simulink model "heli_model2"  (Simulink 10.3)
settings: Solver=ode1  StartTime=0.0  StopTime=100  FixedStep=0.001  RelTol=1e-3
values from neighbouring files (symbols this model uses):
  B_p = 0.0100000    (= 0.01)    [setup_heli_LQR_instructor.m]    (also in setup_heli_LQR_parameters.m)
  B_y = 0.0071428    [setup_heli_LQR_instructor.m]    (also in setup_heli_LQR_parameters.m)
  g = 9.81    [setup_heli_LQR_instructor.m]    (also in setup_heli_LQR_parameters.m)
  h = 0.0139    [setup_heli_LQR_instructor.m]    (also in setup_heli_LQR_parameters.m)
  J_eq_p = 0.0500    (= 0.05)    [setup_heli_LQR_instructor.m]    (also in setup_heli_LQR_parameters.m)
  J_eq_y = 0.0500+0.0039    (= 0.0539)    [setup_heli_LQR_instructor.m]    (also in setup_heli_LQR_parameters.m)
  K_pp = 0.185*0.20962    (= 0.0387797)    [setup_heli_LQR_instructor.m]    (also in setup_heli_LQR_parameters.m)
  K_py = 0.0041362    [setup_heli_LQR_instructor.m]    (also in setup_heli_LQR_parameters.m)
  K_yp = 0.0083316    [setup_heli_LQR_instructor.m]    (also in setup_heli_LQR_parameters.m)
  K_yy = 0.185*0.050271    (= 0.009300135)    [setup_heli_LQR_instructor.m]    (also in setup_heli_LQR_parameters.m)
  Ki = lqr(a,b,Qi,R)    [setup_heli_LQR_instructor.m]
  l_cm = 0.0168    [setup_heli_LQR_instructor.m]    (also in setup_heli_LQR_parameters.m)
  m_heli = 1.326    [setup_heli_LQR_instructor.m]    (also in setup_heli_LQR_parameters.m)
  Rc = 0.0094    [setup_heli_LQR_instructor.m]    (also in setup_heli_LQR_parameters.m)
  SAT_INT_ERR_PITCH = 20    [setup_heli_LQR_instructor.m]    (also in setup_heli_LQR_parameters.m)
  SAT_INT_ERR_YAW = 20    [setup_heli_LQR_instructor.m]    (also in setup_heli_LQR_parameters.m)
  theta_0 = -30*pi/180    (= -0.523598775598)    [setup_heli_LQR_instructor.m]    (also in setup_heli_LQR_parameters.m)
  Tr_p = 1    [setup_heli_LQR_instructor.m]    (also in setup_heli_LQR_parameters.m)
  Tr_y = 1    [setup_heli_LQR_instructor.m]    (also in setup_heli_LQR_parameters.m)
  VMAX_UPM_P = 24    [setup_heli_LQR_instructor.m]    (also in setup_heli_LQR_parameters.m)
  VMAX_UPM_Y = 15    [setup_heli_LQR_instructor.m]    (also in setup_heli_LQR_parameters.m)
undefined symbols (not defined in the file or in its folder): heli_2d_lib, Scopes
libraries: simulink_extras x4
settings Model: Creator=Joseph  LastModifiedBy=Joseph  ExtModeArmWhenConnect=off
settings DataIOCC: LimitDataPoints=on
settings OptimizationCC: BooleanDataType=off  OptimizeBlockIOStorage=off  BufferReuse=off  ExpressionFolding=off  ExpressionDepthLimit=128  LocalBlockOutputs=off  InitFltsAndDblsToZero=on
settings DebuggingCC: SaveWithParameterizedLinksMsg=none  SignalResolutionControl=TryResolveAllWithWarning  SolverPrmCheckMsg=warning  MultiTaskDSMMsg=warning  MultiTaskCondExecSysMsg=none  StateNameClashWarn=none
settings SFSimCC: SimUseLocalCustomCode=on  CustomCodeUndefinedFunction=FilterOut
settings RTWCC: Description=WinCon Target  SystemTargetFile=wincon.tlc  MakeCommand=make_wc  TemplateMakefile=wc_default_tmf  RTWUseLocalCustomCode=on
settings STFCustomTargetCC: TargetFcnLib=ansi_tfl_tmw.mat  ModelReferenceCompliant=off  CPPClassGenCompliant=on  SystemTargetFile=wincon.tlc
settings GRTTargetCC: TargetFcnLib=ansi_tfl_tmw.mat  ModelReferenceCompliant=off  ParMdlRefBuildCompliant=off  CompOptLevelCompliant=off  ConcurrentExecutionCompliant=off  MatFileLogging=off  UseToolchainInfoCompliant=off  ExtMode=on  ExtModeTransport=2  ExtModeMexFile=wc_comm
settings CustomProperty: Value=on
settings ConfigComp: CovExternalEMLEnable=on

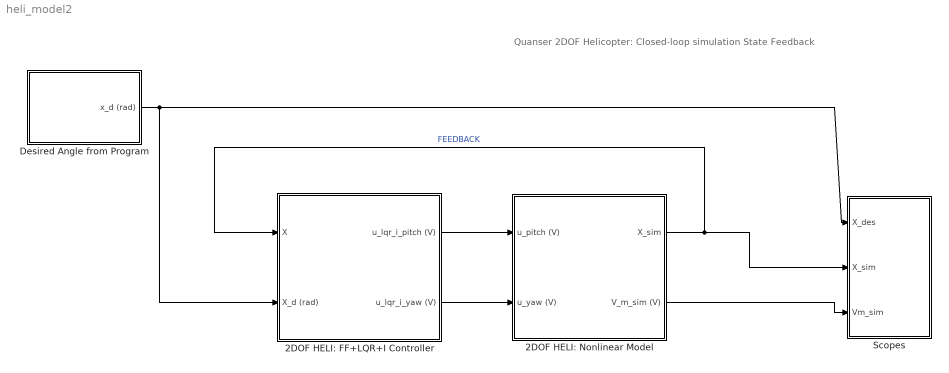
== system heli_model2 ==
  note: Quanser 2DOF Helicopter: Closed-loop simulation
      | State Feedback
  2DOF HELI: FF+LQR+I Controller : Subsystem  AncestorBlock=heli_2d_lib/2DOF HELI: FF+LQR+I Controller
  2DOF HELI: Nonlinear Model : Subsystem  AncestorBlock=heli_2d_lib/2DOF HELI: Nonlinear Model
  Desired Angle from Program : Subsystem
  Scopes : Subsystem  AncestorBlock=heli_2d_lib/Scopes
  wires:
  Desired Angle from Program/1(x_d (rad)) -> Scopes/1(X_des), 2DOF HELI: FF+LQR+I Controller/2(X_d (rad))
  2DOF HELI: FF+LQR+I Controller/1(u_lqr_i_pitch (V)) -> 2DOF HELI: Nonlinear Model/1(u_pitch (V))
  2DOF HELI: FF+LQR+I Controller/2(u_lqr_i_yaw (V)) -> 2DOF HELI: Nonlinear Model/2(u_yaw (V))
  2DOF HELI: Nonlinear Model/1(X_sim) -> Scopes/2(X_sim), 2DOF HELI: FF+LQR+I Controller/1(X)  "FEEDBACK"
  2DOF HELI: Nonlinear Model/2(V_m_sim (V)) -> Scopes/3(Vm_sim)

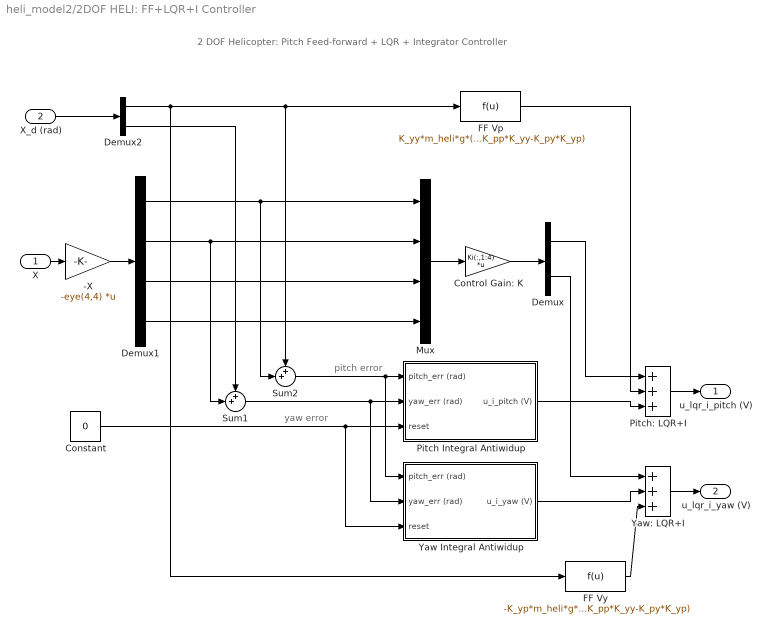
== system heli_model2/2DOF HELI: FF+LQR+I Controller ==
  note: yaw error
  note: pitch error
  note: 2 DOF Helicopter:
      | Pitch Feed-forward + LQR + Integrator Controller
  X : Inport
  X_d (rad) : Inport  Port=2
  -X : Gain  Gain=-eye(4,4)  Multiplication=Matrix(K*u)
  Constant : Constant  Value=0
  Control Gain: K : Gain  Gain=Ki(:,1:4)  Multiplication=Matrix(K*u)
  Demux : Demux  Outputs=2
  Demux1 : Demux
  Demux2 : Demux  Outputs=2
  FF Vp : Fcn  Expr="K_yy*m_heli*g*(h*sin(u[1]) + Rc*cos(u[1]))  /  (K_pp*K_yy-K_py*K_yp)"
  FF Vy : Fcn  Expr="-K_yp*m_heli*g*(h*sin(u[1]) + Rc*cos(u[1]))  /  (K_pp*K_yy-K_py*K_yp)"
  Mux : Mux
  Pitch Integral Antiwidup : Subsystem  AncestorBlock=heli_2d_lib/2DOF HELI: FF+LQR+I Controller/Yaw Integral Antiwidup
  Pitch: LQR+I : Sum  Inputs=+++
  Sum1 : Sum  Inputs=++|
  Sum2 : Sum  Inputs=++|
  Yaw Integral Antiwidup : Subsystem
  Yaw: LQR+I : Sum  Inputs=+++
  u_lqr_i_pitch (V) : Outport
  u_lqr_i_yaw (V) : Outport  Port=2
  wires:
  Constant/1 -> Pitch Integral Antiwidup/3(reset), Yaw Integral Antiwidup/3(reset)
  Demux1/2 -> Sum1/2, Mux/2
  Demux2/2 -> Sum1/1
  Demux2/1 -> Sum2/1, FF Vp/1, FF Vy/1
  X_d (rad)/1 -> Demux2/1
  Yaw Integral Antiwidup/1(u_i_yaw (V)) -> Yaw: LQR+I/2
  Demux/2 -> Yaw: LQR+I/1
  Yaw: LQR+I/1 -> u_lqr_i_yaw (V)/1
  Pitch: LQR+I/1 -> u_lqr_i_pitch (V)/1
  Demux/1 -> Pitch: LQR+I/2
  Pitch Integral Antiwidup/1(u_i_pitch (V)) -> Pitch: LQR+I/3
  FF Vp/1 -> Pitch: LQR+I/1
  Sum2/1 -> Pitch Integral Antiwidup/1(pitch_err (rad)), Yaw Integral Antiwidup/1(pitch_err (rad))
  Demux1/1 -> Sum2/2, Mux/1
  X/1 -> -X/1
  Sum1/1 -> Pitch Integral Antiwidup/2(yaw_err (rad)), Yaw Integral Antiwidup/2(yaw_err (rad))
  -X/1 -> Demux1/1
  Control Gain: K/1 -> Demux/1
  Mux/1 -> Control Gain: K/1
  Demux1/3 -> Mux/3
  Demux1/4 -> Mux/4
  FF Vy/1 -> Yaw: LQR+I/3

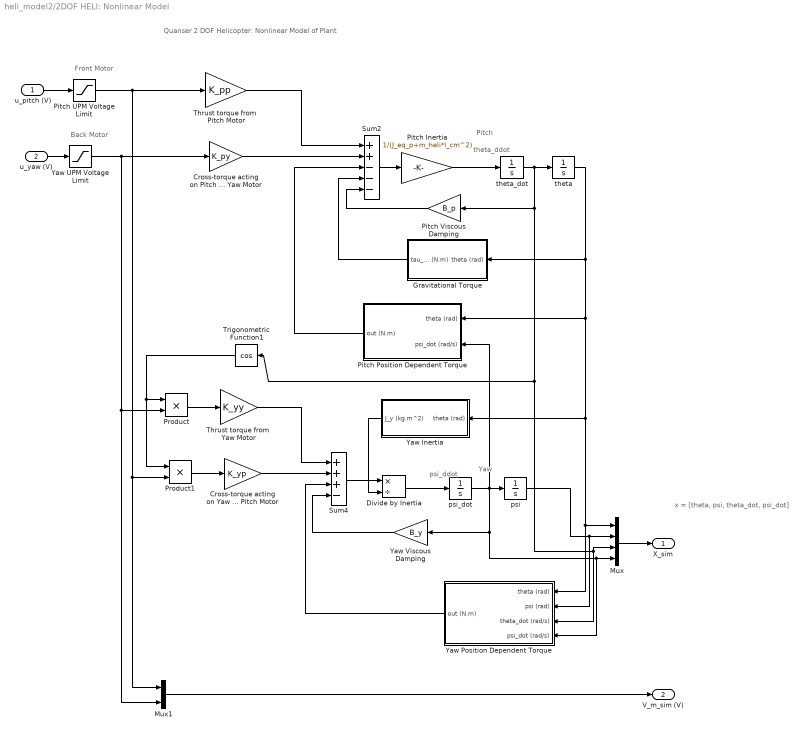
== system heli_model2/2DOF HELI: Nonlinear Model ==
  note: Back Motor
  note: Front Motor
  note: x = [theta, psi, theta_dot, psi_dot]
  note: Quanser 2 DOF Helicopter: Nonlinear Model of Plant
  note: theta_ddot
  note: psi_ddot
  note: Pitch
  note: Yaw
  u_pitch (V) : Inport
  u_yaw (V) : Inport  Port=2
  Cross-torque acting on Pitch  from Yaw Motor : Gain  Gain=K_py
  Cross-torque acting on Yaw  from Pitch Motor : Gain  Gain=K_yp
  Divide by Inertia : Product  Inputs=*/
  Gravitational Torque : Subsystem
  Mux : Mux
  Mux1 : Mux  Inputs=2
  Pitch Inertia : Gain  Gain=1/(J_eq_p+m_heli*l_cm^2)
  Pitch Position Dependent Torque : Subsystem  AncestorBlock=heli_2d_lib/2DOF Helicopter: Nonlinear Model/Yaw Nonlinear Element
  Pitch UPM Voltage Limit : Saturate  UpperLimit=VMAX_UPM_P  LowerLimit=- VMAX_UPM_P
  Pitch Viscous Damping : Gain  Gain=B_p
  Product : Product  RndMeth=Zero
  Product1 : Product  RndMeth=Zero
  Sum2 : Sum  Inputs=++---
  Sum4 : Sum  Inputs=+++-
  Thrust torque from  Pitch Motor : Gain  Gain=K_pp
  Thrust torque from  Yaw Motor : Gain  Gain=K_yy
  Trigonometric Function1 : Trigonometry  Operator=cos  OutputSignalType=real
  Yaw Inertia : Subsystem
  Yaw Position Dependent Torque : Subsystem
  Yaw UPM Voltage Limit : Saturate  UpperLimit=VMAX_UPM_Y  LowerLimit=- VMAX_UPM_Y
  Yaw Viscous Damping : Gain  Gain=B_y
  psi : Integrator
  psi_dot : Integrator
  theta : Integrator  InitialCondition=theta_0  LimitOutput=on  UpperSaturationLimit=40.5*pi/180  LowerSaturationLimit=-40.5*pi/180
  theta_dot : Integrator
  X_sim : Outport
  V_m_sim (V) : Outport  Port=2
  wires:
  Pitch Position Dependent Torque/1(out (N.m)) -> Sum2/3
  Gravitational Torque/1(tau_g (N.m)) -> Sum2/4
  Pitch Viscous Damping/1 -> Sum2/5
  Cross-torque acting on Pitch  from Yaw Motor/1 -> Sum2/2
  Thrust torque from  Pitch Motor/1 -> Sum2/1
  Yaw Inertia/1(J_y (kg.m^2)) -> Divide by Inertia/2
  Divide by Inertia/1 -> psi_dot/1
  Sum4/1 -> Divide by Inertia/1
  Yaw Position Dependent Torque/1(out (N.m)) -> Sum4/3
  Yaw Viscous Damping/1 -> Sum4/4
  psi/1 -> Yaw Position Dependent Torque/2(psi (rad)), Mux/2
  Mux1/1 -> V_m_sim (V)/1
  Yaw UPM Voltage Limit/1 -> Cross-torque acting on Pitch  from Yaw Motor/1, Mux1/2, Product/2
  Pitch UPM Voltage Limit/1 -> Thrust torque from  Pitch Motor/1, Mux1/1, Product1/2
  Mux/1 -> X_sim/1
  theta/1 -> Gravitational Torque/1(theta (rad)), Pitch Position Dependent Torque/1(theta (rad)), Yaw Position Dependent Torque/1(theta (rad)), Mux/1, Yaw Inertia/1(theta (rad))
  Sum2/1 -> Pitch Inertia/1
  Pitch Inertia/1 -> theta_dot/1
  theta_dot/1 -> Pitch Viscous Damping/1, Yaw Position Dependent Torque/3(theta_dot (rad/s)), Mux/3, Trigonometric Function1/1, theta/1
  Thrust torque from  Yaw Motor/1 -> Sum4/1
  Cross-torque acting on Yaw  from Pitch Motor/1 -> Sum4/2
  psi_dot/1 -> Yaw Viscous Damping/1, Yaw Position Dependent Torque/4(psi_dot (rad/s)), Mux/4, Pitch Position Dependent Torque/2(psi_dot (rad/s)), psi/1
  u_pitch (V)/1 -> Pitch UPM Voltage Limit/1
  u_yaw (V)/1 -> Yaw UPM Voltage Limit/1
  Product/1 -> Thrust torque from  Yaw Motor/1
  Trigonometric Function1/1 -> Product/1, Product1/1
  Product1/1 -> Cross-torque acting on Yaw  from Pitch Motor/1

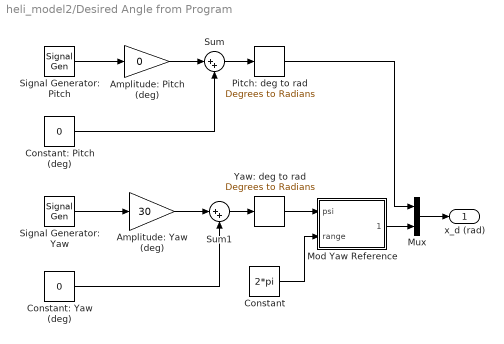
== system heli_model2/Desired Angle from Program ==
  Amplitude: Pitch (deg) : Gain  Gain=0
  Amplitude: Yaw (deg) : Gain  Gain=30
  Constant : Constant  Value=2*pi
  Constant: Pitch (deg) : Constant  Value=0
  Constant: Yaw (deg) : Constant  Value=0
  Mod Yaw Reference : Subsystem
  Mux : Mux  Inputs=2
  Pitch: deg to rad : simulink_extras/Transformations/Degrees to Radians
  Signal Generator: Pitch : SignalGenerator  WaveForm=square  Frequency=1/20
  Signal Generator: Yaw : SignalGenerator  WaveForm=square  Frequency=0.05
  Sum : Sum  Inputs=|++
  Sum1 : Sum  Inputs=|++
  Yaw: deg to rad : simulink_extras/Transformations/Degrees to Radians
  x_d (rad) : Outport
  wires:
  Mux/1 -> x_d (rad)/1
  Constant: Yaw (deg)/1 -> Sum1/2
  Amplitude: Yaw (deg)/1 -> Sum1/1
  Signal Generator: Yaw/1 -> Amplitude: Yaw (deg)/1
  Sum1/1 -> Yaw: deg to rad/1
  Constant: Pitch (deg)/1 -> Sum/2
  Amplitude: Pitch (deg)/1 -> Sum/1
  Signal Generator: Pitch/1 -> Amplitude: Pitch (deg)/1
  Sum/1 -> Pitch: deg to rad/1
  Pitch: deg to rad/1 -> Mux/1
  Mod Yaw Reference/1(mod psi) -> Mux/2
  Yaw: deg to rad/1 -> Mod Yaw Reference/1(psi)
  Constant/1 -> Mod Yaw Reference/2(range)

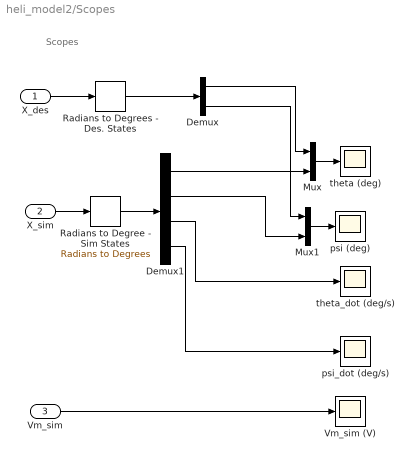
== system heli_model2/Scopes ==
  note: Scopes
  X_des : Inport
  X_sim : Inport  Port=2
  Vm_sim : Inport  Port=3
  Demux : Demux  Outputs=2
  Demux1 : Demux
  Mux : Mux  Inputs=2
  Mux1 : Mux  Inputs=2
  Radians to Degree - Sim States : simulink_extras/Transformations/Radians to Degrees
  Radians to Degrees - Des. States : simulink_extras/Transformations/Radians to Degrees
  Vm_sim (V) : Scope
  psi (deg) : Scope
  psi_dot (deg/s) : Scope
  theta (deg) : Scope
  theta_dot (deg/s) : Scope
  wires:
  Demux1/4 -> psi_dot (deg/s)/1
  Demux1/3 -> theta_dot (deg/s)/1
  Mux1/1 -> psi (deg)/1
  Mux/1 -> theta (deg)/1
  Radians to Degree - Sim States/1 -> Demux1/1
  X_sim/1 -> Radians to Degree - Sim States/1
  X_des/1 -> Radians to Degrees - Des. States/1
  Demux/1 -> Mux/1
  Demux1/1 -> Mux/2
  Demux/2 -> Mux1/1
  Demux1/2 -> Mux1/2
  Radians to Degrees - Des. States/1 -> Demux/1
  Vm_sim/1 -> Vm_sim (V)/1

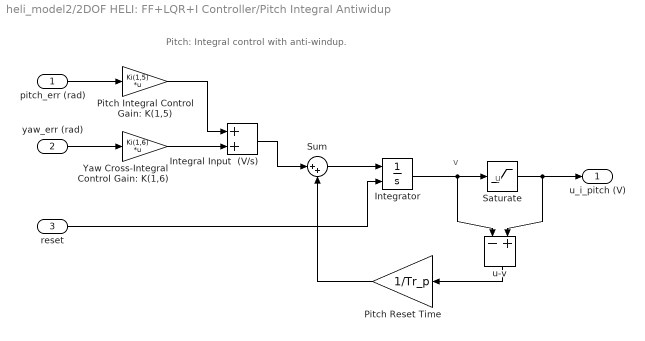
== system heli_model2/2DOF HELI: FF+LQR+I Controller/Pitch Integral Antiwidup ==
  note: Pitch: Integral control with anti-windup.
  note: v
  note: u
  pitch_err (rad) : Inport
  yaw_err (rad) : Inport  Port=2
  reset : Inport  Port=3
  Integral Input  (V/s) : Sum
  Integrator : Integrator  ExternalReset=rising
  Pitch Integral Control Gain: K(1,5) : Gain  Gain=Ki(1,5)  Multiplication=Matrix(K*u)
  Pitch Reset Time : Gain  Gain=1/Tr_p
  Saturate : Saturate  UpperLimit=SAT_INT_ERR_PITCH  LowerLimit=-SAT_INT_ERR_PITCH
  Sum : Sum  Inputs=|++
  Yaw Cross-Integral Control Gain: K(1,6) : Gain  Gain=Ki(1,6)  Multiplication=Matrix(K*u)
  u-v : Sum  Inputs=-+
  u_i_pitch (V) : Outport
  wires:
  Integral Input  (V/s)/1 -> Sum/1
  Yaw Cross-Integral Control Gain: K(1,6)/1 -> Integral Input  (V/s)/2
  Pitch Integral Control Gain: K(1,5)/1 -> Integral Input  (V/s)/1
  yaw_err (rad)/1 -> Yaw Cross-Integral Control Gain: K(1,6)/1
  reset/1 -> Integrator/2
  Pitch Reset Time/1 -> Sum/2
  Sum/1 -> Integrator/1
  u-v/1 -> Pitch Reset Time/1
  Saturate/1 -> u-v/2, u_i_pitch (V)/1
  Integrator/1 -> Saturate/1, u-v/1
  pitch_err (rad)/1 -> Pitch Integral Control Gain: K(1,5)/1

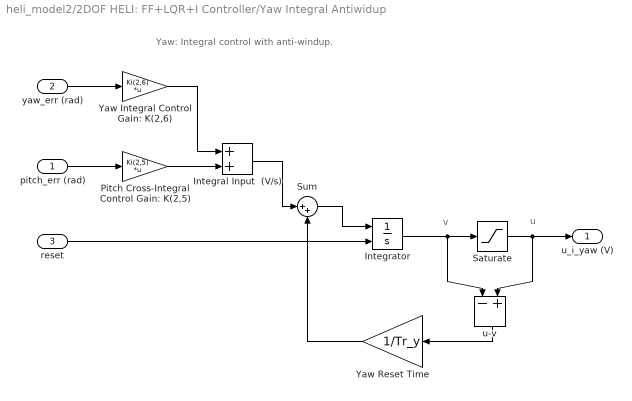
== system heli_model2/2DOF HELI: FF+LQR+I Controller/Yaw Integral Antiwidup ==
  note: Yaw: Integral control with anti-windup.
  note: u
  note: v
  pitch_err (rad) : Inport
  yaw_err (rad) : Inport  Port=2
  reset : Inport  Port=3
  Integral Input  (V/s) : Sum
  Integrator : Integrator  ExternalReset=rising
  Pitch Cross-Integral Control Gain: K(2,5) : Gain  Gain=Ki(2,5)  Multiplication=Matrix(K*u)
  Saturate : Saturate  UpperLimit=SAT_INT_ERR_YAW  LowerLimit=-SAT_INT_ERR_YAW
  Sum : Sum  Inputs=|++
  Yaw Integral Control Gain: K(2,6) : Gain  Gain=Ki(2,6)  Multiplication=Matrix(K*u)
  Yaw Reset Time : Gain  Gain=1/Tr_y
  u-v : Sum  Inputs=-+
  u_i_yaw (V) : Outport
  wires:
  Integral Input  (V/s)/1 -> Sum/1
  Pitch Cross-Integral Control Gain: K(2,5)/1 -> Integral Input  (V/s)/2
  Yaw Integral Control Gain: K(2,6)/1 -> Integral Input  (V/s)/1
  pitch_err (rad)/1 -> Pitch Cross-Integral Control Gain: K(2,5)/1
  reset/1 -> Integrator/2
  yaw_err (rad)/1 -> Yaw Integral Control Gain: K(2,6)/1
  Integrator/1 -> u-v/1, Saturate/1
  Saturate/1 -> u_i_yaw (V)/1, u-v/2
  u-v/1 -> Yaw Reset Time/1
  Sum/1 -> Integrator/1
  Yaw Reset Time/1 -> Sum/2

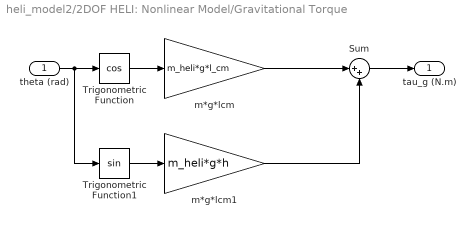
== system heli_model2/2DOF HELI: Nonlinear Model/Gravitational Torque ==
  theta (rad) : Inport
  Sum : Sum  Inputs=|++
  Trigonometric Function : Trigonometry  Operator=cos  OutputSignalType=real
  Trigonometric Function1 : Trigonometry  OutputSignalType=real
  m*g*lcm : Gain  Gain=m_heli*g*l_cm
  m*g*lcm1 : Gain  Gain=m_heli*g*h
  tau_g (N.m) : Outport
  wires:
  theta (rad)/1 -> Trigonometric Function/1, Trigonometric Function1/1
  Trigonometric Function/1 -> m*g*lcm/1
  Trigonometric Function1/1 -> m*g*lcm1/1
  m*g*lcm1/1 -> Sum/2
  m*g*lcm/1 -> Sum/1
  Sum/1 -> tau_g (N.m)/1

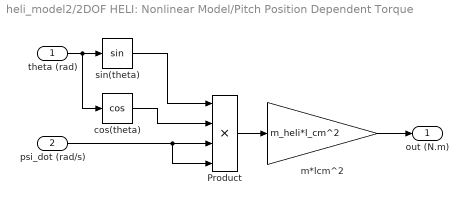
== system heli_model2/2DOF HELI: Nonlinear Model/Pitch Position Dependent Torque ==
  theta (rad) : Inport
  psi_dot (rad/s) : Inport  Port=2
  Product : Product  Inputs=4  RndMeth=Zero
  cos(theta) : Trigonometry  Operator=cos  OutputSignalType=real
  m*lcm^2 : Gain  Gain=m_heli*l_cm^2
  sin(theta) : Trigonometry  OutputSignalType=real
  out (N.m) : Outport
  wires:
  psi_dot (rad/s)/1 -> Product/4, Product/3
  theta (rad)/1 -> cos(theta)/1, sin(theta)/1
  Product/1 -> m*lcm^2/1
  sin(theta)/1 -> Product/1
  cos(theta)/1 -> Product/2
  m*lcm^2/1 -> out (N.m)/1

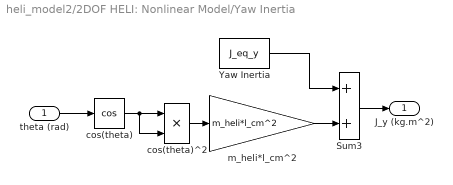
== system heli_model2/2DOF HELI: Nonlinear Model/Yaw Inertia ==
  theta (rad) : Inport
  Sum3 : Sum
  Yaw Inertia : Constant  Value=J_eq_y
  cos(theta) : Trigonometry  Operator=cos  OutputSignalType=real
  cos(theta)^2 : Product  RndMeth=Zero
  m_heli*l_cm^2 : Gain  Gain=m_heli*l_cm^2
  J_y (kg.m^2) : Outport
  wires:
  cos(theta)/1 -> cos(theta)^2/2, cos(theta)^2/1
  Sum3/1 -> J_y (kg.m^2)/1
  theta (rad)/1 -> cos(theta)/1
  m_heli*l_cm^2/1 -> Sum3/2
  Yaw Inertia/1 -> Sum3/1
  cos(theta)^2/1 -> m_heli*l_cm^2/1

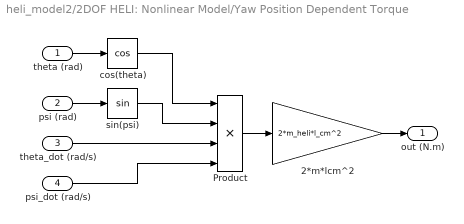
== system heli_model2/2DOF HELI: Nonlinear Model/Yaw Position Dependent Torque ==
  theta (rad) : Inport
  psi (rad) : Inport  Port=2
  theta_dot (rad/s) : Inport  Port=3
  psi_dot (rad/s) : Inport  Port=4
  2*m*lcm^2 : Gain  Gain=2*m_heli*l_cm^2
  Product : Product  Inputs=4  RndMeth=Zero
  cos(theta) : Trigonometry  Operator=cos  OutputSignalType=real
  sin(psi) : Trigonometry  OutputSignalType=real
  out (N.m) : Outport
  wires:
  2*m*lcm^2/1 -> out (N.m)/1
  psi_dot (rad/s)/1 -> Product/4
  theta_dot (rad/s)/1 -> Product/3
  sin(psi)/1 -> Product/2
  cos(theta)/1 -> Product/1
  Product/1 -> 2*m*lcm^2/1
  theta (rad)/1 -> cos(theta)/1
  psi (rad)/1 -> sin(psi)/1

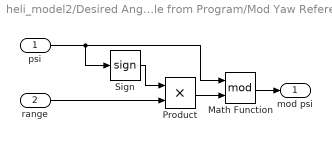
== system heli_model2/Desired Angle from Program/Mod Yaw Reference ==
  psi : Inport
  range : Inport  Port=2
  Math Function : Math  Operator=mod  SignedPower=on  SaturateOnIntegerOverflow=on
  Product : Product  RndMeth=Zero
  Sign : Signum
  mod psi : Outport
  wires:
  Product/1 -> Math Function/2
  Sign/1 -> Product/1
  psi/1 -> Math Function/1, Sign/1
  Math Function/1 -> mod psi/1
  range/1 -> Product/2
